simulink model "usv_twist_controller_generator_002"  (R2021b)
settings: Solver=FixedStepDiscrete  StartTime=0.0  StopTime=inf  FixedStep=twistControllerSampleTime  RelTol=1e-3  EnableMultiTasking=on
PreLoadFcn:
  | % Controller Sample Time
  | twistControllerSampleTime = 0.10;
  | 
  | % Init ros on local ip
  | rosshutdown;
  | localip = 'http://sa:11311';
  | rosinit(localip);
undefined symbols (not defined in the file): DiscIntNeverNeededParam, Left, Right
libraries: robotlib x27, simulink x4, slpidlib x1
settings Model: Creator=altin  LastModifiedBy=sa
settings SolverCC: AllowMultiTaskInputOutput=on  ConcurrentTasks=on  PositivePriorityOrder=on  AutoInsertRateTranBlk=on
settings OptimizationCC: EnhancedBackFolding=on  PassReuseOutputArgsThreshold=0  MaxStackSize=64  OptimizeBlockOrder=speed  DifferentSizesBufferReuse=on  OptimizationCustomize=off
settings DebuggingCC: ParameterTunabilityLossMsg=error
settings HardwareCC: ProdBitPerPointer=32  ProdBitPerSizeT=32  ProdBitPerPtrDiffT=32  ProdLargestAtomicFloat=None  ProdIntDivRoundTo=Undefined  ProdEndianess=Unspecified  ProdWordSize=32  ProdHWDeviceType=Generic->Unspecified (assume 32-bit Generic)
settings ModelReferenceCC: ModelReferenceMinAlgLoopOccurrences=on
settings SFSimCC: MATLABDynamicMemAlloc=off
settings RTWCC: Description=Embedded Coder  SystemTargetFile=ert.tlc  HardwareBoard=Robot Operating System (ROS)  TLCOptions="-aInlineSetEventsForThisBaseRateFcn=TLC_FALSE -aSuppressMultiTaskScheduler=TLC_FALSE  -aRateBasedStepFcn=0"  TemplateMakefile=ert_default_tmf  GenerateReport=on  Toolchain=Catkin  LaunchReport=on  TargetLang=C++
settings CodeAppCC: ForceParamTrailComments=on  OperatorAnnotations=on  StateflowObjectComments=on  MATLABSourceComments=on
settings ERTTargetCC: ERTCustomFileBanners=off  SupportContinuousTime=on  SupportNonInlinedSFcns=on  RemoveResetFunc=off  ModelStepFunctionPrototypeControlCompliant=off  ERTCustomFileTemplate=rostime_codertarget_file_process.tlc

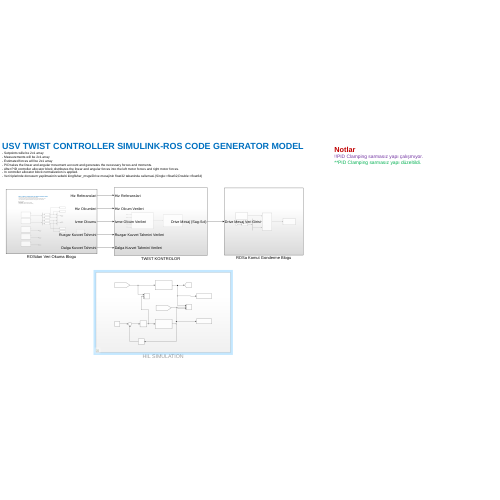
[thumbnail: Simulink's stored preview of the top-level diagram]
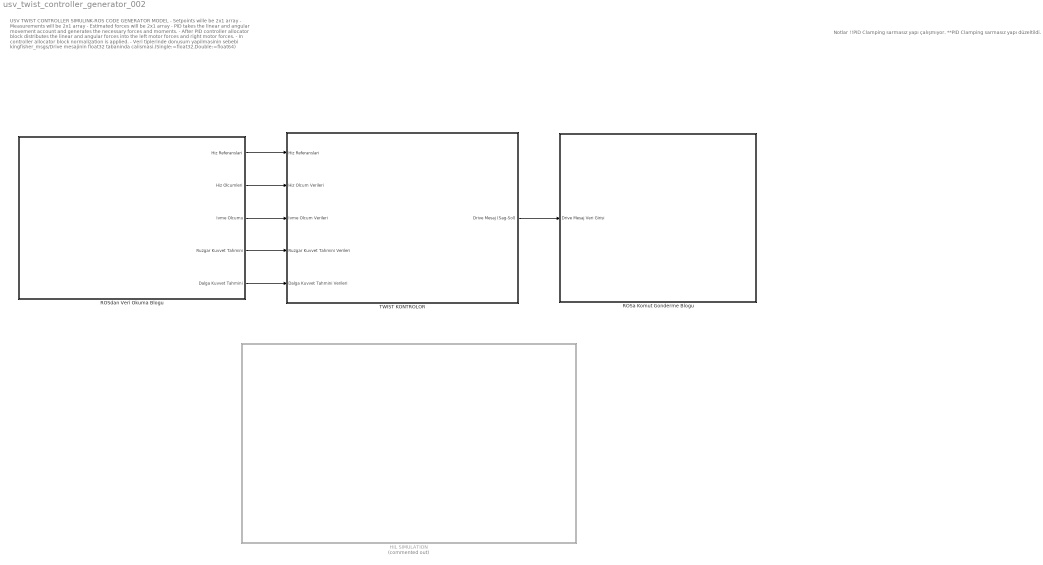
== system usv_twist_controller_generator_002 ==
  note: Notlar
      | !!PID Clamping sarmasız yapı çalışmıyor.
      | **PID Clamping sarmasız yapı düzeltildi.
  note: USV TWIST CONTROLLER SIMULINK-ROS CODE GENERATOR MODEL
      | - Setpoints wille be 2x1 array
      | - Measurements will be 2x1 array
      | - Estimated forces will be 2x1 array
      | - PID takes the linear and angular movement account and generates the necessary forces and moments.
      | - After PID controller allocator block distributes the linear and angular forces into the left motor forces and right motor forces.
      | - In controller allocator block normalization is applied.
      | - Veri tiplerinde donusum yapilmasinin sebebi kingfisher_msgs/Drive mesajinin float32 tabaninda calismasi.(Single:=float32,Double:=float64)
  HIL SIMULATION : Subsystem  Commented=on
  ROSa Komut Gonderme Blogu : Subsystem
  ROSdan Veri Okuma Blogu : Subsystem
  TWIST KONTROLOR : Subsystem
  wires:
  ROSdan Veri Okuma Blogu/1(Hiz Referanslari) -> TWIST KONTROLOR/1(Hiz Referanslari)
  ROSdan Veri Okuma Blogu/2(Hiz Olcumleri) -> TWIST KONTROLOR/2(Hiz Olcum Verileri)
  ROSdan Veri Okuma Blogu/3(Ivme Olcumu) -> TWIST KONTROLOR/3(Ivme Olcum Verileri)
  ROSdan Veri Okuma Blogu/4(Ruzgar Kuvvet Tahmini) -> TWIST KONTROLOR/4(Ruzgar Kuvvet Tahmini Verileri)
  ROSdan Veri Okuma Blogu/5(Dalga Kuvvet Tahmini) -> TWIST KONTROLOR/5(Dalga Kuvvet Tahmini Verileri)
  TWIST KONTROLOR/1(Drive Mesaj (Sag-Sol)) -> ROSa Komut Gonderme Blogu/1(Drive Mesaj Veri Girisi)

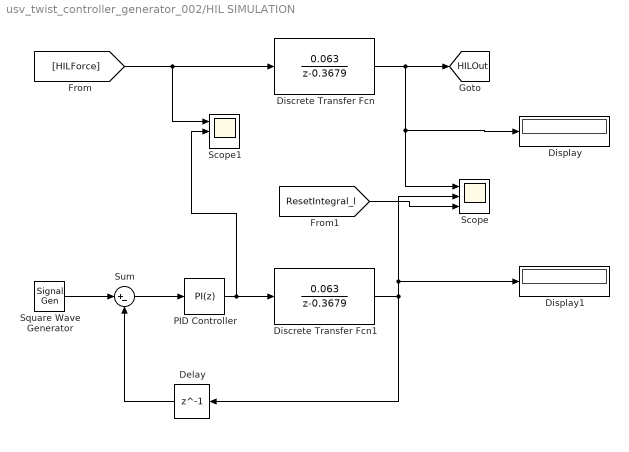
== system usv_twist_controller_generator_002/HIL SIMULATION ==
  Delay : Delay  DelayLength=1
  Discrete Transfer Fcn : DiscreteTransferFcn  Numerator=[0.063]  Denominator=[1 -0.3679]
  Discrete Transfer Fcn1 : DiscreteTransferFcn  Numerator=[0.063]  Denominator=[1 -0.3679]
  Display : Display
  Display1 : Display
  PID Controller : slpidlib/PID Controller  Controller=PI  Form=Parallel  TimeDomain=Discrete-time  UseExternalTs=off  SampleTime=-1  IntegratorMethod=Forward Euler  FilterMethod=Forward Euler  ControllerParametersSource=internal  P=1  I=25  D=0  UseFilter=on  N=100  TunerSelectOption=Transfer Function Based (PID Tuner App)  InitialConditionSource=internal  InitialConditionForIntegrator=0  InitialConditionForFilter=0  DifferentiatorICPrevScaledInput=0  ExternalReset=none  TrackingMode=off  Kt=1  LimitOutput=off  SatLimitsSource=internal  UpperSaturationLimit=inf  LowerSaturationLimit=-inf  LinearizeAsGain=on  AntiWindupMode=none  Kb=1  POutMin=[]  POutMax=[]  IOutMin=[]  IOutMax=[]  DOutMin=[]  DOutMax=[]  NOutMin=[]  NOutMax=[]  SumOutMin=[]  SumOutMax=[]  SaturationOutMin=[]  SaturationOutMax=[]  PParamMin=[]  PParamMax=[]  IParamMin=[]  IParamMax=[]  DParamMin=[]  DParamMax=[]  NParamMin=[]  NParamMax=[]  KbParamMin=[]  KbParamMax=[]  KtParamMin=[]  KtParamMax=[]  KbOutMin=[]  KbOutMax=[]  KtOutMin=[]  KtOutMax=[]  IntegratorOutMin=[]  IntegratorOutMax=[]  FilterOutMin=[]  FilterOutMax=[]  SumI1OutMin=[]  SumI1OutMax=[]  SumI2OutMin=[]  SumI2OutMax=[]  SumI3OutMin=[]  SumI3OutMax=[]  SumI4OutMin=[]  SumI4OutMax=[]  SumDOutMin=[]  SumDOutMax=[]  DifferentiatorOutMin=[]  DifferentiatorOutMax=[]  FilterDiffOutCoefMin=[]  FilterDiffOutCoefMax=[]  ReciprocalOutMin=[]  ReciprocalOutMax=[]  SumDenOutMin=[]  SumDenOutMax=[]  SumNumOutMin=[]  SumNumOutMax=[]  DivideOutMin=[]  DivideOutMax=[]  UdiffTsProdOutMin=[]  UdiffTsProdOutMax=[]  NTsProdOutMin=[]  NTsProdOutMax=[]  UintegralTsProdOutMin=[]  UintegralTsProdOutMax=[]  UngainTsProdOutMin=[]  UngainTsProdOutMax=[]  IntegratorContinuousStateAttributes=''  IntegratorStateMustResolveToSignalObject=off  IntegratorRTWStateStorageClass=Auto  FilterContinuousStateAttributes=''  FilterStateMustResolveToSignalObject=off  FilterRTWStateStorageClass=Auto  ParallelPVariant=InternalParameters  IdealPVariant=Disabled  IVariant=InternalParameters  DVariant=Disabled  IntegratorVariant=Discrete  SatVariant=Disabled  AWVariant=Passthrough  PCopyVariant=Disabled  TRVariant=Disabled  FdbkBlocksVariant=Forward  IdealPFdbkVariant=Disabled  SatFdbkVariant=Disabled  DerivativeFilterVariant=Disabled  NVariant=Disabled  NCopyVariant=Disabled_SignalSpec  FilterICVariant=Disabled  IntegratorICVariant=InternalICs  ExternalResetVariant=Disabled  TRSumVariant=Passthrough  SumFdbkVariant=Disabled  SumVariant=Sum_PI  TsampFilterVariant=InternalTs  TsampNgainVariant=Passthrough  TsampIntegralVariant=Passthrough  ExternalSaturationOutDataTypeStr=Inherit: Same as second input
  Scope : Scope  NumInputPorts=3
  Scope1 : Scope  NumInputPorts=3
  Square Wave Generator : SignalGenerator  WaveForm=square  Frequency=0.8  Units=rad/sec
  Sum : Sum  Inputs=|+-
  tag scope: HILOut=global
  wires:
  [HILForce] -> Scope1/1, Discrete Transfer Fcn/1
  Discrete Transfer Fcn/1 -> Display/1, Scope/1, [HILOut]
  PID Controller/1 -> Scope1/2, Discrete Transfer Fcn1/1
  Sum/1 -> PID Controller/1
  Discrete Transfer Fcn1/1 -> Delay/1, Display1/1, Scope/2
  Delay/1 -> Sum/2
  Square Wave Generator/1 -> Sum/1
  [ResetIntegral_l] -> Scope/3

== system usv_twist_controller_generator_002/ROSa Komut Gonderme Blogu ==
  Drive Mesaj Veri Girisi : Inport
  Bus Assignment : BusAssignment  AssignedSignals=Right,Left
  Data Type Conversion : DataTypeConversion  OutDataTypeStr=single
  Demux : Demux  Outputs=2
  MOSA Drive Mesaj Tanimi : robotlib/Blank Message  messageClass=Message  entityType=kingfisher_msgs/Drive  messageType=kingfisher_msgs/Drive  SampleTime=inf  legacyBusStruct=off
  MOSA Komut Topigi : robotlib/Publish  topicSource=Select from ROS network  topic=/MOSA1/mosa_cmd_vel_mux/input/joy  messageType=kingfisher_msgs/Drive  legacyBusStruct=off  messageQueueLength=1
  wires:
  Drive Mesaj Veri Girisi/1 -> Data Type Conversion/1
  Bus Assignment/1 -> MOSA Komut Topigi/1
  MOSA Drive Mesaj Tanimi/1 -> Bus Assignment/1
  Data Type Conversion/1 -> Demux/1
  Demux/1 -> Bus Assignment/2
  Demux/2 -> Bus Assignment/3

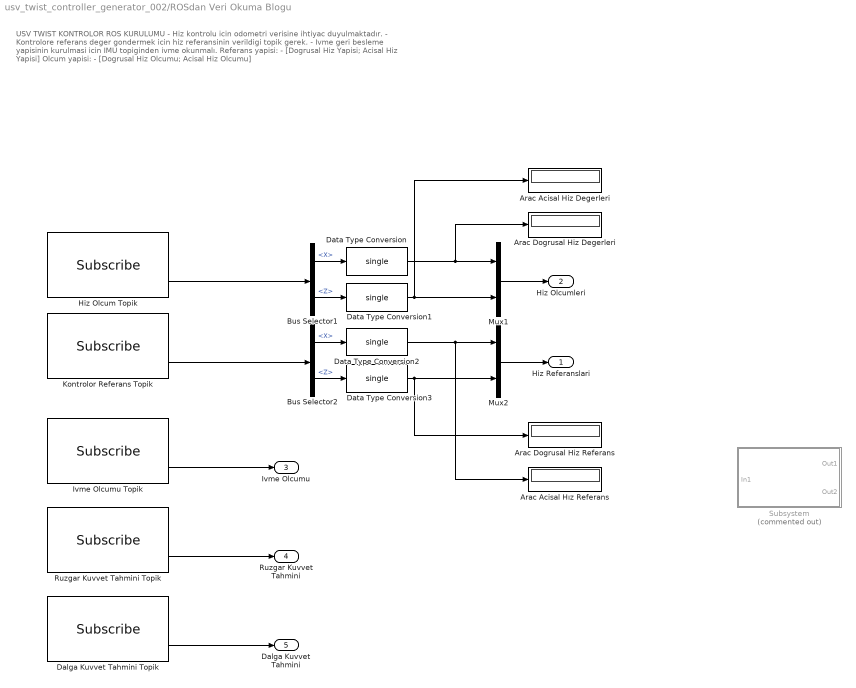
== system usv_twist_controller_generator_002/ROSdan Veri Okuma Blogu ==
  note: USV TWIST KONTROLOR ROS KURULUMU
      | - Hiz kontrolu icin odometri verisine ihtiyac duyulmaktadır.
      | - Kontrolore referans deger gondermek icin hiz referansinin verildigi topik gerek.
      | - Ivme geri besleme yapisinin kurulmasi icin IMU topiginden ivme okunmalı.
      |
      | Referans yapisi:
      | - [Dogrusal Hiz Yapisi; Acisal Hiz Yapisi]
      | Olcum yapisi:
      | - [Dogrusal Hiz Olcumu; Acisal Hiz Olcumu]
  Arac Acisal Hiz Degerleri : Display
  Arac Acisal Hız Referans : Display
  Arac Dogrusal Hiz Degerleri : Display
  Arac Dogrusal Hiz Referans : Display
  Bus Selector1 : BusSelector  OutputSignals=Twist.Twist.Linear.X,Twist.Twist.Angular.Z
  Bus Selector2 : BusSelector  OutputSignals=Linear.X,Angular.Z
  Dalga Kuvvet Tahmini Topik : robotlib/Subscribe  topicSource=Select from ROS network  topic=/my_topic  messageType=geometry_msgs/Point  SampleTime=-1  legacyBusStruct=off  messageQueueLength=1
  Data Type Conversion{,1..3} (4 alike) : DataTypeConversion  OutDataTypeStr=single
  Hiz Olcum Topik : robotlib/Subscribe  topicSource=Select from ROS network  topic=/MOSA1/gx5/nav/odom  messageType=nav_msgs/Odometry  SampleTime=-1  legacyBusStruct=off  messageQueueLength=1
  Ivme Olcumu Topik : robotlib/Subscribe  topicSource=Select from ROS network  topic=/my_topic  messageType=geometry_msgs/Point  SampleTime=-1  legacyBusStruct=off  messageQueueLength=1
  Kontrolor Referans Topik : robotlib/Subscribe  topicSource=Specify your own  topic=/MOSA1/velocity_setpoints  messageType=geometry_msgs/Twist  SampleTime=-1  legacyBusStruct=off  messageQueueLength=1
  Mux1 : Mux  Inputs=2
  Mux2 : Mux  Inputs=2
  Ruzgar Kuvvet Tahmini Topik : robotlib/Subscribe  topicSource=Select from ROS network  topic=/my_topic  messageType=geometry_msgs/Point  SampleTime=-1  legacyBusStruct=off  messageQueueLength=1
  Subsystem : Subsystem  Commented=on
  Hiz Referanslari : Outport
  Hiz Olcumleri : Outport  Port=2
  Ivme Olcumu : Outport  Port=3
  Ruzgar Kuvvet Tahmini : Outport  Port=4
  Dalga Kuvvet Tahmini : Outport  Port=5
  wires:
  Hiz Olcum Topik/2 -> Bus Selector1/1
  Bus Selector1/1 -> Data Type Conversion/1  "<X>"
  Data Type Conversion/1 -> Arac Dogrusal Hiz Degerleri/1, Mux1/1
  Data Type Conversion1/1 -> Arac Acisal Hiz Degerleri/1, Mux1/2
  Bus Selector1/2 -> Data Type Conversion1/1  "<Z>"
  Kontrolor Referans Topik/2 -> Bus Selector2/1
  Data Type Conversion2/1 -> Arac Acisal Hız Referans/1, Mux2/1
  Data Type Conversion3/1 -> Arac Dogrusal Hiz Referans/1, Mux2/2
  Bus Selector2/2 -> Data Type Conversion3/1  "<Z>"
  Bus Selector2/1 -> Data Type Conversion2/1  "<X>"
  Mux1/1 -> Hiz Olcumleri/1
  Mux2/1 -> Hiz Referanslari/1
  Ivme Olcumu Topik/2 -> Ivme Olcumu/1
  Ruzgar Kuvvet Tahmini Topik/2 -> Ruzgar Kuvvet Tahmini/1
  Dalga Kuvvet Tahmini Topik/2 -> Dalga Kuvvet Tahmini/1

== system usv_twist_controller_generator_002/TWIST KONTROLOR ==
  Hiz Referanslari : Inport
  Hiz Olcum Verileri : Inport  Port=2
  Ivme Olcum Verileri : Inport  Port=3
  Ruzgar Kuvvet Tahmini Verileri : Inport  Port=4
  Dalga Kuvvet Tahmini Verileri : Inport  Port=5
  KONTROLOR AYRISTIRICI (SAG_SOL MOTOR ICIN) : Subsystem
  TWIST PID KONTROLOR : Subsystem
  Drive Mesaj (Sag-Sol) : Outport
  wires:
  TWIST PID KONTROLOR/1(Kontrolor Cikisi) -> KONTROLOR AYRISTIRICI (SAG_SOL MOTOR ICIN)/1(Controller Out)
  Hiz Referanslari/1 -> TWIST PID KONTROLOR/1(Referanslar)
  Hiz Olcum Verileri/1 -> TWIST PID KONTROLOR/2(Hiz Olcumleri)
  Ivme Olcum Verileri/1 -> TWIST PID KONTROLOR/3(Ivme Olcumleri)
  Ruzgar Kuvvet Tahmini Verileri/1 -> TWIST PID KONTROLOR/4(Ruzgar Kuvvet Tahmini)
  Dalga Kuvvet Tahmini Verileri/1 -> TWIST PID KONTROLOR/5(Dalga Kuvvet Tahmini)
  KONTROLOR AYRISTIRICI (SAG_SOL MOTOR ICIN)/1(Drive Message Data) -> Drive Mesaj (Sag-Sol)/1

== system usv_twist_controller_generator_002/ROSdan Veri Okuma Blogu/Subsystem ==
  In1 : Inport
  Mux : Mux  Inputs=2
  Mux3 : Mux  Inputs=2
  Square Wave Generator : SignalGenerator  WaveForm=square  Frequency=0.8  Units=rad/sec
  Out1 : Outport
  Out2 : Outport  Port=2
  wires:
  Mux3/1 -> Out2/1
  Mux/1 -> Out1/1
  [HILOut] -> Mux3/1
  In1/1 -> Mux3/2
  Square Wave Generator/1 -> Mux/2, Mux/1

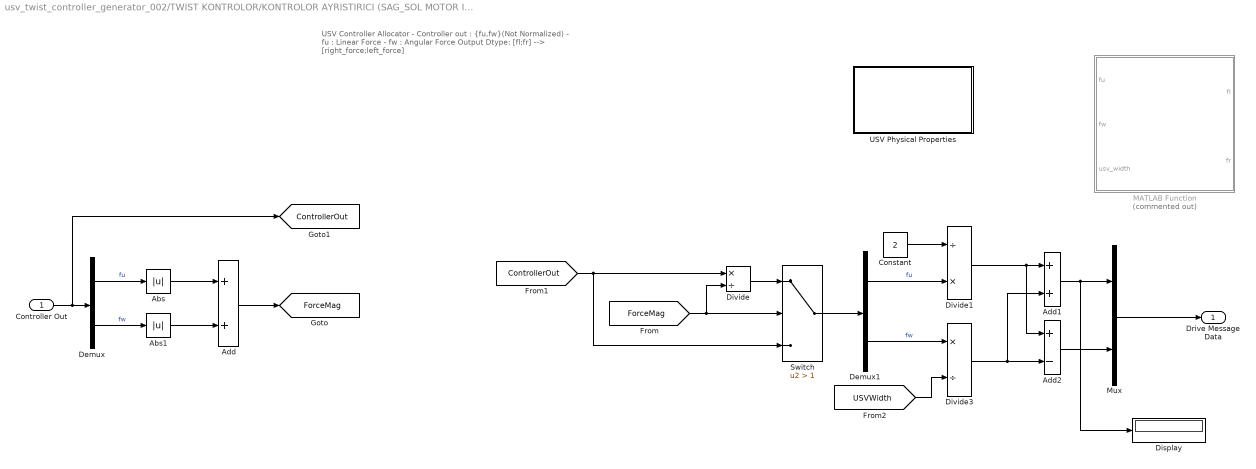
== system usv_twist_controller_generator_002/TWIST KONTROLOR/KONTROLOR AYRISTIRICI (SAG_SOL MOTOR ICIN) ==
  note: USV Controller Allocator
      | - Controller out : {fu,fw}(Not Normalized)
      | - fu : Linear Force
      | - fw : Angular Force
      |
      | Output Dtype:
      | [fl;fr] --> [right_force;left_force]
  Controller Out : Inport
  Abs : Abs
  Abs1 : Abs
  Add : Sum
  Add1 : Sum
  Add2 : Sum  Inputs=+-
  Constant : Constant  Value=2
  Demux : Demux  Outputs=2
  Demux1 : Demux  Outputs=2
  Display : Display
  Divide : Product  Inputs=*/
  Divide1 : Product  Inputs=/*
  Divide3 : Product  Inputs=*/
  MATLAB Function : MATLAB Function  Commented=on  TreatAsAtomicUnit=on
  Mux : Mux  Inputs=2
  Switch : Switch  Criteria=u2 > Threshold  Threshold=1
  USV Physical Properties : Subsystem
  Drive Message Data : Outport
  tag scope: ControllerOut=global, ForceMag=global
  wires:
  Controller Out/1 -> [ControllerOut], Demux/1
  Demux/1 -> Abs/1  "fu"
  Demux/2 -> Abs1/1  "fw"
  Abs1/1 -> Add/2
  Abs/1 -> Add/1
  Add/1 -> [ForceMag]
  [ForceMag] -> Divide/2, Switch/2
  [ControllerOut] -> Switch/3, Divide/1
  Divide/1 -> Switch/1
  Switch/1 -> Demux1/1
  Mux/1 -> Drive Message Data/1
  Demux1/2 -> Divide3/1  "fw"
  [USVWidth] -> Divide3/2
  Demux1/1 -> Divide1/2  "fu"
  Constant/1 -> Divide1/1
  Divide1/1 -> Add2/1, Add1/1
  Divide3/1 -> Add1/2, Add2/2
  Add1/1 -> Display/1, Mux/1
  Add2/1 -> Mux/2

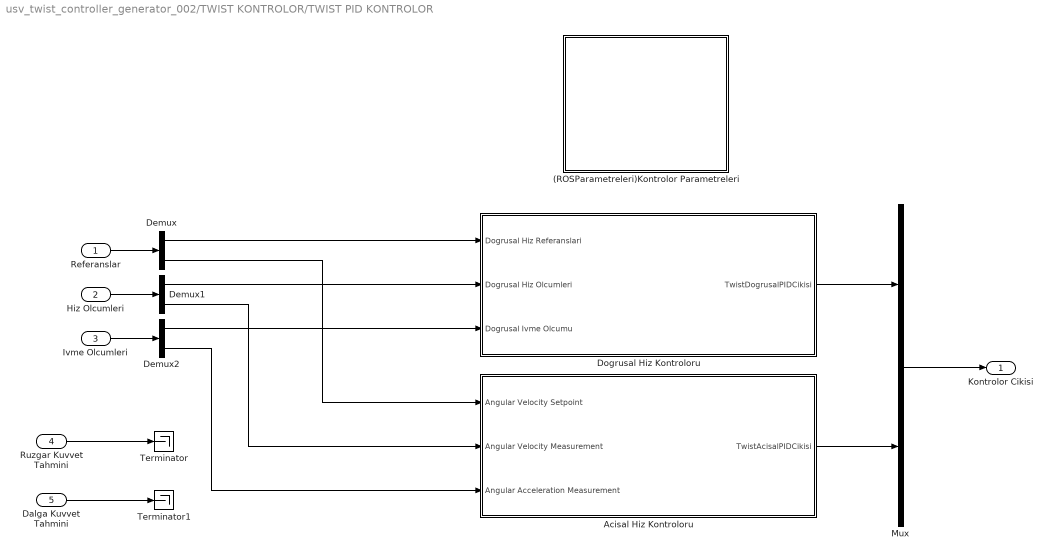
== system usv_twist_controller_generator_002/TWIST KONTROLOR/TWIST PID KONTROLOR ==
  Referanslar : Inport
  Hiz Olcumleri : Inport  Port=2
  Ivme Olcumleri : Inport  Port=3
  Ruzgar Kuvvet Tahmini : Inport  Port=4
  Dalga Kuvvet Tahmini : Inport  Port=5
  (ROSParametreleri)Kontrolor Parametreleri : Subsystem
  Acisal Hiz Kontroloru : Subsystem
  Demux : Demux  Outputs=2
  Demux1 : Demux  Outputs=2
  Demux2 : Demux  Outputs=2
  Dogrusal Hiz Kontroloru : Subsystem
  Mux : Mux  Inputs=2
  Terminator : Terminator
  Terminator1 : Terminator
  Kontrolor Cikisi : Outport
  wires:
  Referanslar/1 -> Demux/1
  Demux/1 -> Dogrusal Hiz Kontroloru/1(Dogrusal Hiz Referanslari)
  Demux/2 -> Acisal Hiz Kontroloru/1(Angular Velocity Setpoint)
  Ruzgar Kuvvet Tahmini/1 -> Terminator/1
  Dalga Kuvvet Tahmini/1 -> Terminator1/1
  Ivme Olcumleri/1 -> Demux2/1
  Hiz Olcumleri/1 -> Demux1/1
  Demux1/1 -> Dogrusal Hiz Kontroloru/2(Dogrusal Hiz Olcumleri)
  Demux1/2 -> Acisal Hiz Kontroloru/2(Angular Velocity Measurement)
  Demux2/1 -> Dogrusal Hiz Kontroloru/3(Dogrusal Ivme Olcumu)
  Demux2/2 -> Acisal Hiz Kontroloru/3(Angular Acceleration Measurement)
  Dogrusal Hiz Kontroloru/1(TwistDogrusalPIDCikisi) -> Mux/1
  Acisal Hiz Kontroloru/1(TwistAcisalPIDCikisi) -> Mux/2
  Mux/1 -> Kontrolor Cikisi/1

== system usv_twist_controller_generator_002/TWIST KONTROLOR/KONTROLOR AYRISTIRICI (SAG_SOL MOTOR ICIN)/USV Physical Properties ==
  Data Type Conversion : DataTypeConversion  OutDataTypeStr=single
  Display : Display
  Twist Angular Ag : robotlib/Get Parameter  ParameterSource=Select from ROS network  ParameterName=/MOSA1/USVWidth  ParameterType=double  ParameterMaxArrayLength=16  ParameterInitialValue=0.0  SampleTime=-1  ShowErrorCodeOutput=on  ModelName=usv_twist_controller_generator_002  BlockId=ParamGet_usv_twist_controller_generator_002_280
      settings: SourceProductBaseCode=RR
  tag scope: USVWidth=global
  wires:
  Twist Angular Ag/1 -> Data Type Conversion/1
  Data Type Conversion/1 -> Display/1, [USVWidth]

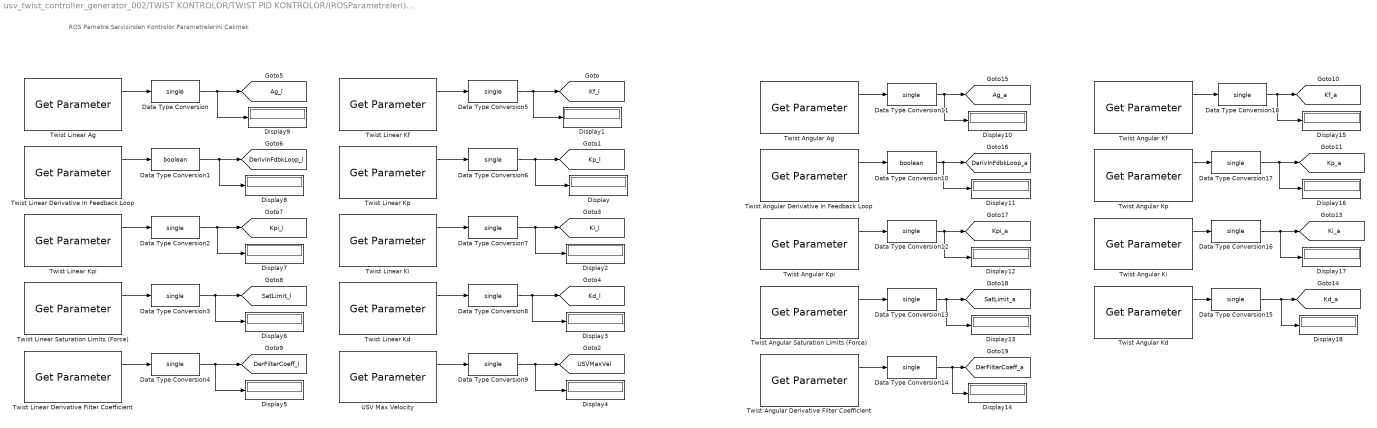
== system usv_twist_controller_generator_002/TWIST KONTROLOR/TWIST PID KONTROLOR/(ROSParametreleri)Kontrolor Parametreleri ==
  note: ROS Pametre Servisinden Kontrolor Parametrelerini Cekmek
  Data Type Conversion{,2..9,11..18} (17 alike) : DataTypeConversion  OutDataTypeStr=single
  Data Type Conversion1 : DataTypeConversion  OutDataTypeStr=boolean
  Data Type Conversion10 : DataTypeConversion  OutDataTypeStr=boolean
  Display{,1..18} (19 alike) : Display
  Twist Angular Ag : robotlib/Get Parameter  ParameterSource=Select from ROS network  ParameterName=/MOSA1/AgAngular  ParameterType=double  ParameterMaxArrayLength=16  ParameterInitialValue=0.0  SampleTime=-1  ShowErrorCodeOutput=on  ModelName=usv_twist_controller_generator_002  BlockId=ParamGet_usv_twist_controller_generator_002_169
      settings: SourceProductBaseCode=RR
  Twist Angular Derivative Filter Coefficient : robotlib/Get Parameter  ParameterSource=Select from ROS network  ParameterName=/MOSA1/PIDDerivativeFilterCoefficientAngular  ParameterType=double  ParameterMaxArrayLength=16  ParameterInitialValue=0.0  SampleTime=-1  ShowErrorCodeOutput=on  ModelName=usv_twist_controller_generator_002  BlockId=ParamGet_usv_twist_controller_generator_002_170
      settings: SourceProductBaseCode=RR
  Twist Angular Derivative In Feedback Loop : robotlib/Get Parameter  ParameterSource=Select from ROS network  ParameterName=/MOSA1/DerivativeInFeedbackAngular  ParameterType=int32  ParameterMaxArrayLength=16  ParameterInitialValue=0.0  SampleTime=-1  ShowErrorCodeOutput=on  ModelName=usv_twist_controller_generator_002  BlockId=ParamGet_usv_twist_controller_generator_002_171
      settings: SourceProductBaseCode=RR
  Twist Angular Kd : robotlib/Get Parameter  ParameterSource=Select from ROS network  ParameterName=/MOSA1/KdAngular  ParameterType=double  ParameterMaxArrayLength=16  ParameterInitialValue=0.0  SampleTime=-1  ShowErrorCodeOutput=on  ModelName=usv_twist_controller_generator_002  BlockId=ParamGet_usv_twist_controller_generator_002_172
      settings: SourceProductBaseCode=RR
  Twist Angular Kf : robotlib/Get Parameter  ParameterSource=Select from ROS network  ParameterName=/MOSA1/KfAngular  ParameterType=double  ParameterMaxArrayLength=16  ParameterInitialValue=0.0  SampleTime=-1  ShowErrorCodeOutput=on  ModelName=usv_twist_controller_generator_002  BlockId=ParamGet_usv_twist_controller_generator_002_173
      settings: SourceProductBaseCode=RR
  Twist Angular Ki : robotlib/Get Parameter  ParameterSource=Select from ROS network  ParameterName=/MOSA1/KiAngular  ParameterType=double  ParameterMaxArrayLength=16  ParameterInitialValue=0.0  SampleTime=-1  ShowErrorCodeOutput=on  ModelName=usv_twist_controller_generator_002  BlockId=ParamGet_usv_twist_controller_generator_002_174
      settings: SourceProductBaseCode=RR
  Twist Angular Kp : robotlib/Get Parameter  ParameterSource=Select from ROS network  ParameterName=/MOSA1/KpAngular  ParameterType=double  ParameterMaxArrayLength=16  ParameterInitialValue=0.0  SampleTime=-1  ShowErrorCodeOutput=on  ModelName=usv_twist_controller_generator_002  BlockId=ParamGet_usv_twist_controller_generator_002_175
      settings: SourceProductBaseCode=RR
  Twist Angular Kpi : robotlib/Get Parameter  ParameterSource=Select from ROS network  ParameterName=/MOSA1/KpiAngular  ParameterType=double  ParameterMaxArrayLength=16  ParameterInitialValue=0.0  SampleTime=-1  ShowErrorCodeOutput=on  ModelName=usv_twist_controller_generator_002  BlockId=ParamGet_usv_twist_controller_generator_002_176
      settings: SourceProductBaseCode=RR
  Twist Angular Saturation Limits (Force) : robotlib/Get Parameter  ParameterSource=Select from ROS network  ParameterName=/MOSA1/ForceSaturationAngular  ParameterType=double  ParameterMaxArrayLength=16  ParameterInitialValue=0.0  SampleTime=-1  ShowErrorCodeOutput=on  ModelName=usv_twist_controller_generator_002  BlockId=ParamGet_usv_twist_controller_generator_002_177
      settings: SourceProductBaseCode=RR
  Twist Linear Ag : robotlib/Get Parameter  ParameterSource=Select from ROS network  ParameterName=/MOSA1/AgLinear  ParameterType=double  ParameterMaxArrayLength=16  ParameterInitialValue=0.0  SampleTime=-1  ShowErrorCodeOutput=on  ModelName=usv_twist_controller_generator_002  BlockId=ParamGet_usv_twist_controller_generator_002_9
      settings: SourceProductBaseCode=RR
  Twist Linear Derivative Filter Coefficient : robotlib/Get Parameter  ParameterSource=Select from ROS network  ParameterName=/MOSA1/PIDDerivativeFilterCoefficientLinear  ParameterType=double  ParameterMaxArrayLength=16  ParameterInitialValue=0.0  SampleTime=-1  ShowErrorCodeOutput=on  ModelName=usv_twist_controller_generator_002  BlockId=ParamGet_usv_twist_controller_generator_002_50
      settings: SourceProductBaseCode=RR
  Twist Linear Derivative In Feedback Loop : robotlib/Get Parameter  ParameterSource=Select from ROS network  ParameterName=/MOSA1/DerivativeInFeedbackLinear  ParameterType=int32  ParameterMaxArrayLength=16  ParameterInitialValue=0.0  SampleTime=-1  ShowErrorCodeOutput=on  ModelName=usv_twist_controller_generator_002  BlockId=ParamGet_usv_twist_controller_generator_002_10
      settings: SourceProductBaseCode=RR
  Twist Linear Kd : robotlib/Get Parameter  ParameterSource=Select from ROS network  ParameterName=/MOSA1/KdLinear  ParameterType=double  ParameterMaxArrayLength=16  ParameterInitialValue=0.0  SampleTime=-1  ShowErrorCodeOutput=on  ModelName=usv_twist_controller_generator_002  BlockId=ParamGet_usv_twist_controller_generator_002_8
      settings: SourceProductBaseCode=RR
  Twist Linear Kf : robotlib/Get Parameter  ParameterSource=Select from ROS network  ParameterName=/MOSA1/KfLinear  ParameterType=double  ParameterMaxArrayLength=16  ParameterInitialValue=0.0  SampleTime=-1  ShowErrorCodeOutput=on  ModelName=usv_twist_controller_generator_002  BlockId=ParamGet_usv_twist_controller_generator_002_11
      settings: SourceProductBaseCode=RR
  Twist Linear Ki : robotlib/Get Parameter  ParameterSource=Select from ROS network  ParameterName=/MOSA1/KiLinear  ParameterType=double  ParameterMaxArrayLength=16  ParameterInitialValue=0.0  SampleTime=-1  ShowErrorCodeOutput=on  ModelName=usv_twist_controller_generator_002  BlockId=ParamGet_usv_twist_controller_generator_002_7
      settings: SourceProductBaseCode=RR
  Twist Linear Kp : robotlib/Get Parameter  ParameterSource=Select from ROS network  ParameterName=/MOSA1/KpLinear  ParameterType=double  ParameterMaxArrayLength=16  ParameterInitialValue=0.0  SampleTime=-1  ShowErrorCodeOutput=on  ModelName=usv_twist_controller_generator_002  BlockId=ParamGet_usv_twist_controller_generator_002_3
      settings: SourceProductBaseCode=RR
  Twist Linear Kpi : robotlib/Get Parameter  ParameterSource=Select from ROS network  ParameterName=/MOSA1/KpiLinear  ParameterType=double  ParameterMaxArrayLength=16  ParameterInitialValue=0.0  SampleTime=-1  ShowErrorCodeOutput=on  ModelName=usv_twist_controller_generator_002  BlockId=ParamGet_usv_twist_controller_generator_002_12
      settings: SourceProductBaseCode=RR
  Twist Linear Saturation Limits (Force) : robotlib/Get Parameter  ParameterSource=Select from ROS network  ParameterName=/MOSA1/ForceSaturationLinear  ParameterType=double  ParameterMaxArrayLength=16  ParameterInitialValue=0.0  SampleTime=-1  ShowErrorCodeOutput=on  ModelName=usv_twist_controller_generator_002  BlockId=ParamGet_usv_twist_controller_generator_002_13
      settings: SourceProductBaseCode=RR
  USV Max Velocity : robotlib/Get Parameter  ParameterSource=Select from ROS network  ParameterName=/MOSA1/USVMaxVelocity  ParameterType=double  ParameterMaxArrayLength=16  ParameterInitialValue=0.0  SampleTime=-1  ShowErrorCodeOutput=on  ModelName=usv_twist_controller_generator_002  BlockId=ParamGet_usv_twist_controller_generator_002_21
      settings: SourceProductBaseCode=RR
  tag scope: Ag_a=global, Ag_l=global, DerFilterCoeff_a=global, DerFilterCoeff_l=global, DerivInFdbkLoop_a=global, DerivInFdbkLoop_l=global, Kd_a=global, Kd_l=global, Kf_a=global, Kf_l=global, Ki_a=global, Ki_l=global, Kp_a=global, Kp_l=global, Kpi_a=global, Kpi_l=global, SatLimit_a=global, SatLimit_l=global, USVMaxVel=global
  wires:
  Twist Angular Ki/1 -> Data Type Conversion16/1
  Twist Angular Kp/1 -> Data Type Conversion17/1
  Twist Angular Kd/1 -> Data Type Conversion15/1
  Twist Angular Kf/1 -> Data Type Conversion18/1
  Twist Linear Ag/1 -> Data Type Conversion/1
  Data Type Conversion/1 -> Display9/1, [Ag_l]
  Twist Linear Derivative In Feedback Loop/1 -> Data Type Conversion1/1
  Data Type Conversion1/1 -> Display8/1, [DerivInFdbkLoop_l]
  Data Type Conversion2/1 -> Display7/1, [Kpi_l]
  Twist Linear Kpi/1 -> Data Type Conversion2/1
  Twist Linear Saturation Limits (Force)/1 -> Data Type Conversion3/1
  Data Type Conversion3/1 -> Display6/1, [SatLimit_l]
  Twist Linear Derivative Filter Coefficient/1 -> Data Type Conversion4/1
  Data Type Conversion4/1 -> Display5/1, [DerFilterCoeff_l]
  Twist Linear Kf/1 -> Data Type Conversion5/1
  Data Type Conversion5/1 -> Display1/1, [Kf_l]
  Twist Linear Kp/1 -> Data Type Conversion6/1
  Data Type Conversion6/1 -> Display/1, [Kp_l]
  Twist Linear Ki/1 -> Data Type Conversion7/1
  Data Type Conversion7/1 -> Display2/1, [Ki_l]
  Twist Linear Kd/1 -> Data Type Conversion8/1
  USV Max Velocity/1 -> Data Type Conversion9/1
  Data Type Conversion9/1 -> Display4/1, [USVMaxVel]
  Data Type Conversion8/1 -> Display3/1, [Kd_l]
  Twist Angular Derivative In Feedback Loop/1 -> Data Type Conversion10/1
  Data Type Conversion10/1 -> Display11/1, [DerivInFdbkLoop_a]
  Twist Angular Ag/1 -> Data Type Conversion11/1
  Data Type Conversion11/1 -> Display10/1, [Ag_a]
  Twist Angular Kpi/1 -> Data Type Conversion12/1
  Data Type Conversion12/1 -> Display12/1, [Kpi_a]
  Twist Angular Saturation Limits (Force)/1 -> Data Type Conversion13/1
  Data Type Conversion13/1 -> Display13/1, [SatLimit_a]
  Data Type Conversion14/1 -> Display14/1, [DerFilterCoeff_a]
  Twist Angular Derivative Filter Coefficient/1 -> Data Type Conversion14/1
  Data Type Conversion18/1 -> Display15/1, [Kf_a]
  Data Type Conversion17/1 -> Display16/1, [Kp_a]
  Data Type Conversion16/1 -> Display17/1, [Ki_a]
  Data Type Conversion15/1 -> Display18/1, [Kd_a]

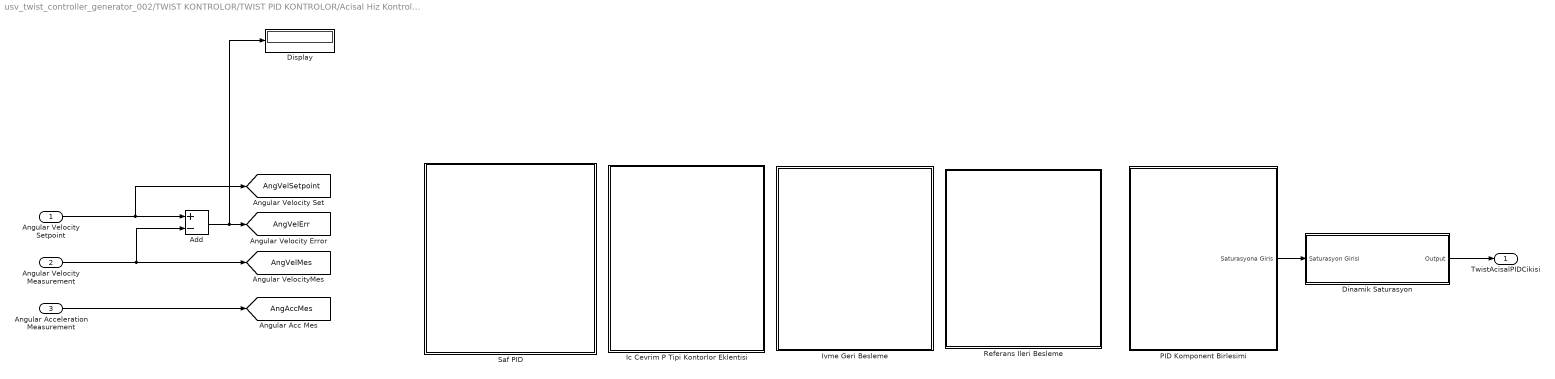
== system usv_twist_controller_generator_002/TWIST KONTROLOR/TWIST PID KONTROLOR/Acisal Hiz Kontroloru ==
  Angular Velocity Setpoint : Inport
  Angular Velocity Measurement : Inport  Port=2
  Angular Acceleration Measurement : Inport  Port=3
  Add : Sum  Inputs=+-
  Dinamik Saturasyon : Subsystem
  Display : Display
  Ic Cevrim P Tipi Kontorlor Eklentisi : Subsystem
  Ivme Geri Besleme : Subsystem
  PID Komponent Birlesimi : Subsystem
  Referans Ileri Besleme : Subsystem
  Saf PID : Subsystem
  TwistAcisalPIDCikisi : Outport
  tag scope: AngAccMes=global, AngVelErr=global, AngVelMes=global, AngVelSetpoint=global
  wires:
  PID Komponent Birlesimi/1(Saturasyona Giris) -> Dinamik Saturasyon/1(Saturasyon Girisi)
  Angular Acceleration Measurement/1 -> [AngAccMes]
  Angular Velocity Measurement/1 -> [AngVelMes], Add/2
  Angular Velocity Setpoint/1 -> [AngVelSetpoint], Add/1
  Add/1 -> Display/1, [AngVelErr]
  Dinamik Saturasyon/1(Output) -> TwistAcisalPIDCikisi/1

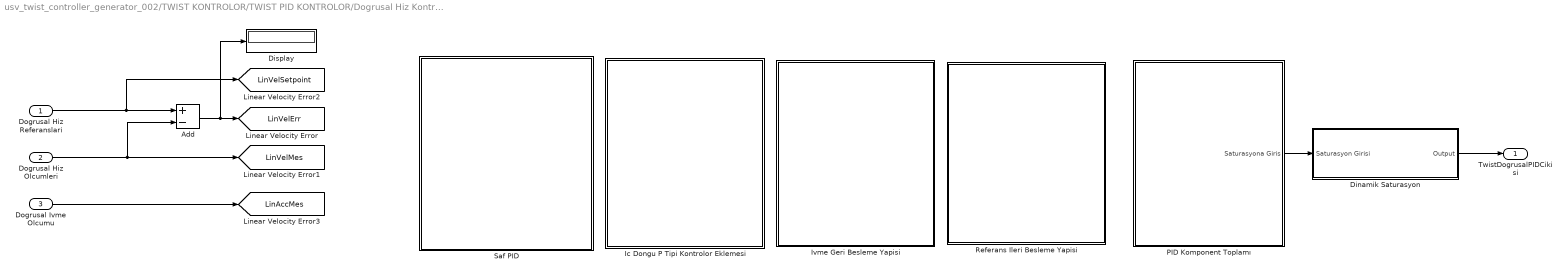
== system usv_twist_controller_generator_002/TWIST KONTROLOR/TWIST PID KONTROLOR/Dogrusal Hiz Kontroloru ==
  Dogrusal Hiz Referanslari : Inport
  Dogrusal Hiz Olcumleri : Inport  Port=2
  Dogrusal Ivme Olcumu : Inport  Port=3
  Add : Sum  Inputs=+-
  Dinamik Saturasyon : Subsystem
  Display : Display
  Ic Dongu P Tipi Kontrolor Eklemesi : Subsystem
  Ivme Geri Besleme Yapisi : Subsystem
  PID Komponent Toplamı : Subsystem
  Referans Ileri Besleme Yapisi : Subsystem
  Saf PID : Subsystem
  TwistDogrusalPIDCikisi : Outport
  tag scope: LinAccMes=global, LinVelErr=global, LinVelMes=global, LinVelSetpoint=global
  wires:
  Dogrusal Hiz Referanslari/1 -> [LinVelSetpoint], Add/1
  Dogrusal Hiz Olcumleri/1 -> [LinVelMes], Add/2
  Add/1 -> Display/1, [LinVelErr]
  Dogrusal Ivme Olcumu/1 -> [LinAccMes]
  Dinamik Saturasyon/1(Output) -> TwistDogrusalPIDCikisi/1
  PID Komponent Toplamı/1(Saturasyona Giris) -> Dinamik Saturasyon/1(Saturasyon Girisi)

== system usv_twist_controller_generator_002/TWIST KONTROLOR/TWIST PID KONTROLOR/Acisal Hiz Kontroloru/Dinamik Saturasyon ==
  Saturasyon Girisi : Inport
  Add : Sum  Inputs=+-
  Compare To Zero : simulink/Logic and Bit Operations/Compare To Zero  relop=>  OutDataTypeStr=boolean
  Display : Display
  Display1 : Display
  Saturation Dynamic : simulink/Discontinuities/Saturation Dynamic  OutMin=[]  OutMax=[]  OutDataTypeStr=single  OutputDataTypeScalingMode=single  OutDataType=fixdt(1, 16)  OutScaling=2^-10  DoSatur=off
  Unary Minus : UnaryMinus
  Output : Outport
  tag scope: ResetIntegral_a=global
  wires:
  Unary Minus/1 -> Saturation Dynamic/3
  [SatLimit_a] -> Saturation Dynamic/1, Unary Minus/1
  Saturasyon Girisi/1 -> Add/2, Saturation Dynamic/2
  Saturation Dynamic/1 -> Display1/1, Output/1, Add/1
  Add/1 -> Compare To Zero/1
  Compare To Zero/1 -> Display/1, [ResetIntegral_a]

== system usv_twist_controller_generator_002/TWIST KONTROLOR/TWIST PID KONTROLOR/Acisal Hiz Kontroloru/Ic Cevrim P Tipi Kontorlor Eklentisi ==
  note: Inner-Loop P Controller
  Add3 : Sum  Inputs=+-
  Product4 : Product
  tag scope: PIDWInnerLoopP_a=global
  wires:
  [AngVelMes] -> Add3/2
  [Kpi_a] -> Product4/2
  Product4/1 -> [PIDWInnerLoopP_a]
  [PIDOut_a] -> Add3/1
  Add3/1 -> Product4/1

== system usv_twist_controller_generator_002/TWIST KONTROLOR/TWIST PID KONTROLOR/Acisal Hiz Kontroloru/Ivme Geri Besleme ==
  Product : Product
  tag scope: AccFdbkOut_a=global
  wires:
  [AngAccMes] -> Product/1
  [Ag_a] -> Product/2
  Product/1 -> [AccFdbkOut_a]

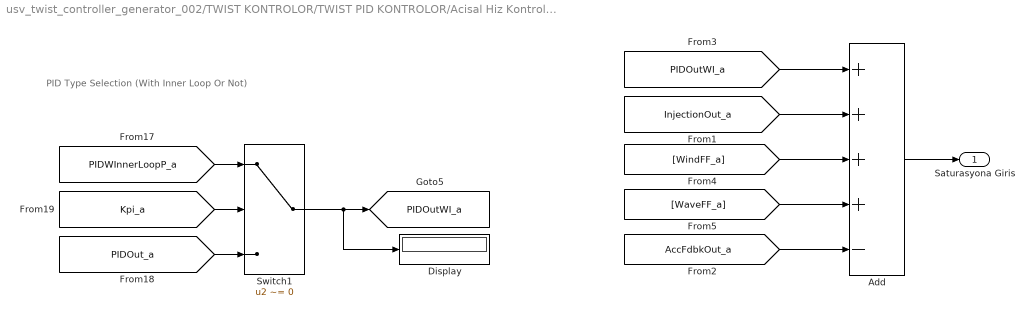
== system usv_twist_controller_generator_002/TWIST KONTROLOR/TWIST PID KONTROLOR/Acisal Hiz Kontroloru/PID Komponent Birlesimi ==
  note: PID Type Selection (With Inner Loop Or Not)
  Add : Sum  Inputs=++++-
  Display : Display
  Switch1 : Switch  Criteria=u2 ~= 0
  Saturasyona Giris : Outport
  tag scope: PIDOutWI_a=global
  wires:
  [PIDOut_a] -> Switch1/3
  [PIDWInnerLoopP_a] -> Switch1/1
  Switch1/1 -> Display/1, [PIDOutWI_a]
  [Kpi_a] -> Switch1/2
  [AccFdbkOut_a] -> Add/5
  [WaveFF_a] -> Add/4
  [WindFF_a] -> Add/3
  [InjectionOut_a] -> Add/2
  [PIDOutWI_a] -> Add/1
  Add/1 -> Saturasyona Giris/1

== system usv_twist_controller_generator_002/TWIST KONTROLOR/TWIST PID KONTROLOR/Acisal Hiz Kontroloru/Referans Ileri Besleme ==
  note: Reference Injection (Velocity Feedforward)
  Product5 : Product
  tag scope: InjectionOut_a=global
  wires:
  [AngVelSetpoint] -> Product5/1
  Product5/1 -> [InjectionOut_a]
  [Kf_a] -> Product5/2

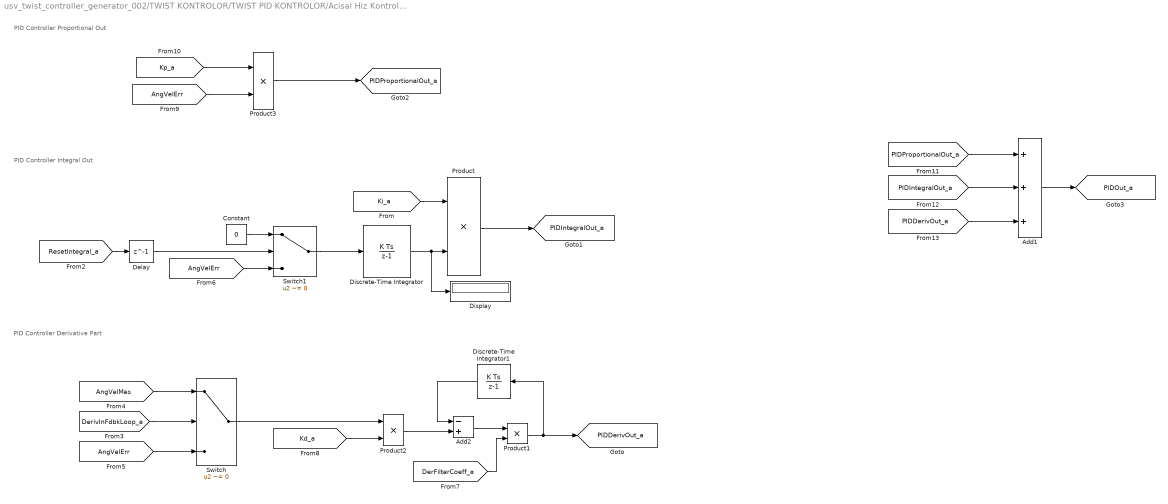
== system usv_twist_controller_generator_002/TWIST KONTROLOR/TWIST PID KONTROLOR/Acisal Hiz Kontroloru/Saf PID ==
  note: PID Controller Derivative Part
  note: PID Controller Integral Out
  note: PID Controller Proportional Out
  Add1 : Sum  Inputs=+++
  Add2 : Sum  Inputs=-+
  Constant : Constant  Value=0  OutDataTypeStr=single
  Delay : Delay  DelayLength=1
  Discrete-Time Integrator : DiscreteIntegrator  SampleTime=twistControllerSampleTime  ICPrevOutput=DiscIntNeverNeededParam  ICPrevScaledInput=DiscIntNeverNeededParam
  Discrete-Time Integrator1 : DiscreteIntegrator  SampleTime=twistControllerSampleTime  ICPrevOutput=DiscIntNeverNeededParam  ICPrevScaledInput=DiscIntNeverNeededParam
  Display : Display
  Product{,1..3} (4 alike) : Product
  Switch : Switch  Criteria=u2 ~= 0
  Switch1 : Switch  Criteria=u2 ~= 0
  tag scope: PIDDerivOut_a=global, PIDIntegralOut_a=global, PIDOut_a=global, PIDProportionalOut_a=global
  wires:
  Product/1 -> [PIDIntegralOut_a]
  Product3/1 -> [PIDProportionalOut_a]
  Product1/1 -> [PIDDerivOut_a], Discrete-Time Integrator1/1
  [DerivInFdbkLoop_a] -> Switch/2
  [AngVelMes] -> Switch/1
  Product2/1 -> Add2/2
  [Kd_a] -> Product2/2
  Switch/1 -> Product2/1
  [Kp_a] -> Product3/1
  [AngVelErr] -> Product3/2
  [DerFilterCoeff_a] -> Product1/2
  Discrete-Time Integrator/1 -> Display/1, Product/2
  Add2/1 -> Product1/1
  [Ki_a] -> Product/1
  [AngVelErr] -> Switch/3
  Discrete-Time Integrator1/1 -> Add2/1
  [PIDIntegralOut_a] -> Add1/2
  Add1/1 -> [PIDOut_a]
  [PIDDerivOut_a] -> Add1/3
  [PIDProportionalOut_a] -> Add1/1
  [ResetIntegral_a] -> Delay/1
  Switch1/1 -> Discrete-Time Integrator/1
  Delay/1 -> Switch1/2
  Constant/1 -> Switch1/1
  [AngVelErr] -> Switch1/3

== system usv_twist_controller_generator_002/TWIST KONTROLOR/TWIST PID KONTROLOR/Dogrusal Hiz Kontroloru/Dinamik Saturasyon ==
  Saturasyon Girisi : Inport
  Add : Sum  Inputs=+-
  Compare To Zero : simulink/Logic and Bit Operations/Compare To Zero  relop=>  OutDataTypeStr=boolean
  Saturation Dynamic : simulink/Discontinuities/Saturation Dynamic  OutMin=[]  OutMax=[]  OutDataTypeStr=single  OutputDataTypeScalingMode=single  OutDataType=fixdt(1, 16)  OutScaling=2^-10  DoSatur=off
  Scope : Scope  NumInputPorts=2
  Unary Minus : UnaryMinus
  Output : Outport
  tag scope: ResetIntegral_l=global
  wires:
  Unary Minus/1 -> Saturation Dynamic/3
  [SatLimit_l] -> Saturation Dynamic/1, Unary Minus/1
  Saturasyon Girisi/1 -> Add/2, Saturation Dynamic/2
  Saturation Dynamic/1 -> Scope/1, Output/1, Add/1
  Compare To Zero/1 -> Scope/2, [ResetIntegral_l]
  Add/1 -> Compare To Zero/1

== system usv_twist_controller_generator_002/TWIST KONTROLOR/TWIST PID KONTROLOR/Dogrusal Hiz Kontroloru/Ic Dongu P Tipi Kontrolor Eklemesi ==
  note: Inner-Loop P Controller
  Add3 : Sum  Inputs=+-
  Product4 : Product
  tag scope: PIDWInnerLoopP_l=global
  wires:
  [LinVelMes] -> Add3/2
  [Kpi_l] -> Product4/2
  Product4/1 -> [PIDWInnerLoopP_l]
  [PIDOut_l] -> Add3/1
  Add3/1 -> Product4/1

== system usv_twist_controller_generator_002/TWIST KONTROLOR/TWIST PID KONTROLOR/Dogrusal Hiz Kontroloru/Ivme Geri Besleme Yapisi ==
  Product : Product
  tag scope: AccFdbkOut_l=global
  wires:
  [LinAccMes] -> Product/1
  [Ag_l] -> Product/2
  Product/1 -> [AccFdbkOut_l]

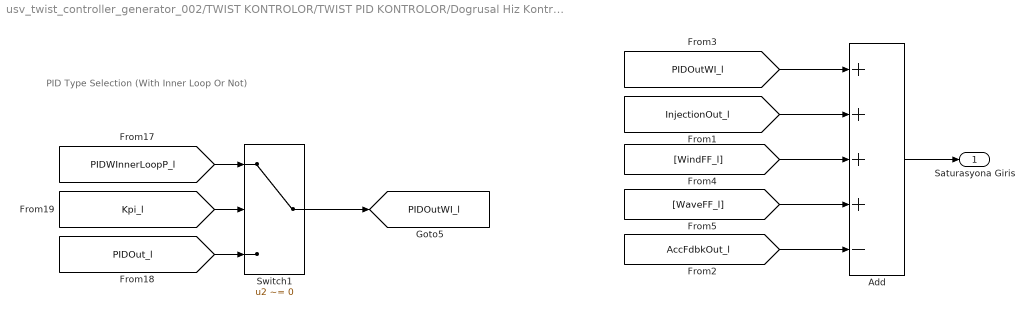
== system usv_twist_controller_generator_002/TWIST KONTROLOR/TWIST PID KONTROLOR/Dogrusal Hiz Kontroloru/PID Komponent Toplamı ==
  note: PID Type Selection (With Inner Loop Or Not)
  Add : Sum  Inputs=++++-
  Switch1 : Switch  Criteria=u2 ~= 0
  Saturasyona Giris : Outport
  tag scope: PIDOutWI_l=global
  wires:
  [PIDOut_l] -> Switch1/3
  [PIDWInnerLoopP_l] -> Switch1/1
  Switch1/1 -> [PIDOutWI_l]
  [Kpi_l] -> Switch1/2
  [AccFdbkOut_l] -> Add/5
  [WaveFF_l] -> Add/4
  [WindFF_l] -> Add/3
  [InjectionOut_l] -> Add/2
  [PIDOutWI_l] -> Add/1
  Add/1 -> Saturasyona Giris/1

== system usv_twist_controller_generator_002/TWIST KONTROLOR/TWIST PID KONTROLOR/Dogrusal Hiz Kontroloru/Referans Ileri Besleme Yapisi ==
  note: Reference Injection (Velocity Feedforward)
  Product5 : Product
  tag scope: InjectionOut_l=global
  wires:
  [LinVelSetpoint] -> Product5/1
  Product5/1 -> [InjectionOut_l]
  [Kf_l] -> Product5/2

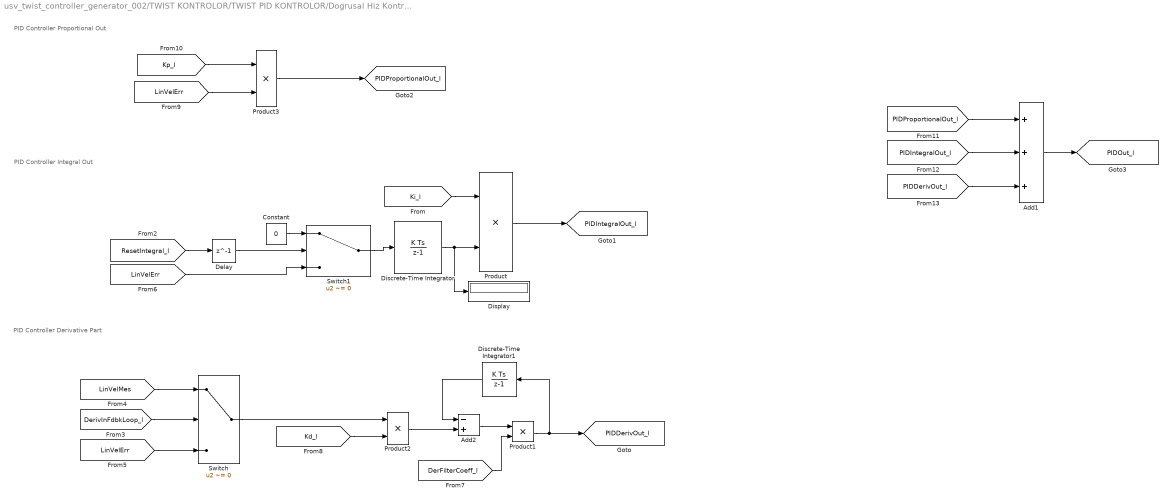
== system usv_twist_controller_generator_002/TWIST KONTROLOR/TWIST PID KONTROLOR/Dogrusal Hiz Kontroloru/Saf PID ==
  note: PID Controller Derivative Part
  note: PID Controller Integral Out
  note: PID Controller Proportional Out
  Add1 : Sum  Inputs=+++
  Add2 : Sum  Inputs=-+
  Constant : Constant  Value=0  OutDataTypeStr=single
  Delay : Delay  DelayLength=1
  Discrete-Time Integrator : DiscreteIntegrator  SampleTime=twistControllerSampleTime  ICPrevOutput=DiscIntNeverNeededParam  ICPrevScaledInput=DiscIntNeverNeededParam
  Discrete-Time Integrator1 : DiscreteIntegrator  SampleTime=twistControllerSampleTime  ICPrevOutput=DiscIntNeverNeededParam  ICPrevScaledInput=DiscIntNeverNeededParam
  Display : Display
  Product{,1..3} (4 alike) : Product
  Switch : Switch  Criteria=u2 ~= 0
  Switch1 : Switch  Criteria=u2 ~= 0
  tag scope: PIDDerivOut_l=global, PIDIntegralOut_l=global, PIDOut_l=global, PIDProportionalOut_l=global
  wires:
  Product/1 -> [PIDIntegralOut_l]
  Product3/1 -> [PIDProportionalOut_l]
  Product1/1 -> [PIDDerivOut_l], Discrete-Time Integrator1/1
  [DerivInFdbkLoop_l] -> Switch/2
  [LinVelMes] -> Switch/1
  Product2/1 -> Add2/2
  [Kd_l] -> Product2/2
  Switch/1 -> Product2/1
  [Kp_l] -> Product3/1
  [LinVelErr] -> Product3/2
  [DerFilterCoeff_l] -> Product1/2
  Discrete-Time Integrator/1 -> Display/1, Product/2
  Add2/1 -> Product1/1
  [Ki_l] -> Product/1
  [LinVelErr] -> Switch/3
  Discrete-Time Integrator1/1 -> Add2/1
  [PIDIntegralOut_l] -> Add1/2
  Add1/1 -> [PIDOut_l]
  [PIDDerivOut_l] -> Add1/3
  [PIDProportionalOut_l] -> Add1/1
  [ResetIntegral_l] -> Delay/1
  Delay/1 -> Switch1/2
  Switch1/1 -> Discrete-Time Integrator/1
  Constant/1 -> Switch1/1
  [LinVelErr] -> Switch1/3

== matlab function usv_twist_controller_generator_002/TWIST KONTROLOR/KONTROLOR AYRISTIRICI (SAG_SOL MOTOR ICIN)/MATLAB Function ==
  data: fu input; fl output; fw input; fr output; usv_width input
function [fl,fr] = controller_allocator(fu,fw,usv_width)

% Calculate the right and left motor necessary forces
fr = (fu/2)+(fw/usv_width);
fl = (fu/2)-(fw/usv_width);
